simulink model "prystupalab4_si"  (R2023b)
settings: Solver=VariableStepAuto  StartTime=0.0  StopTime=10.0  RelTol=1e-3
values from neighbouring files (symbols this model uses):
  a0 = 9    [prystupalab4.m]
  b = 4    [prystupalab4.m]
  d0 = 0    [prystupalab4.m]
  du = 0    [prystupalab4.m]
  k = 1/a1    (= 0.166666666667)    [prystupalab4.m]
  t0 = 0    [prystupalab4.m]
  u0 = 5    [prystupalab4.m]
  x0 = x(i)    [prystupalab4.m]
settings Model: Creator=Adam  LastModifiedBy=Adam

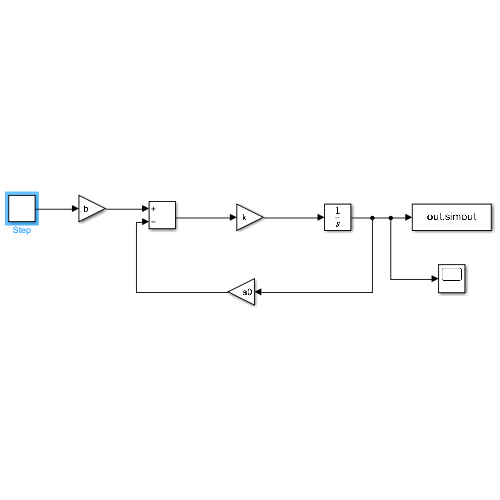
[thumbnail: Simulink's stored preview of the top-level diagram]
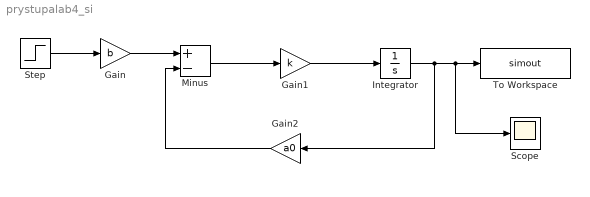
== system prystupalab4_si ==
  Gain : Gain  Gain=b
  Gain1 : Gain  Gain=k
  Gain2 : Gain  Gain=a0
  Integrator : Integrator  InitialCondition=x0
  Minus : Sum  Inputs=+-
  Scope : Scope
  Step : Step  Time=t0  Before=d0  After=d0+u0  SampleTime=du
  To Workspace : ToWorkspace  VariableName=simout  SampleTime=-1
  wires:
  Step/1 -> Gain/1
  Gain/1 -> Minus/1
  Minus/1 -> Gain1/1
  Gain1/1 -> Integrator/1
  Integrator/1 -> Scope/1, To Workspace/1, Gain2/1
  Gain2/1 -> Minus/2
